simulink model "RefModel_TaskOutput_tmp_backup"  (R2015b)
settings: configuration reference "CenterOutReachConfigSet" (kept outside this file)
undefined symbols (not defined in the file or in its folder): SimulinkParameter_TunableNote
settings Model: Creator=djoshea  LastModifiedBy=shenoylab
settings ConfigSetRef: SourceLocation=Base Workspace

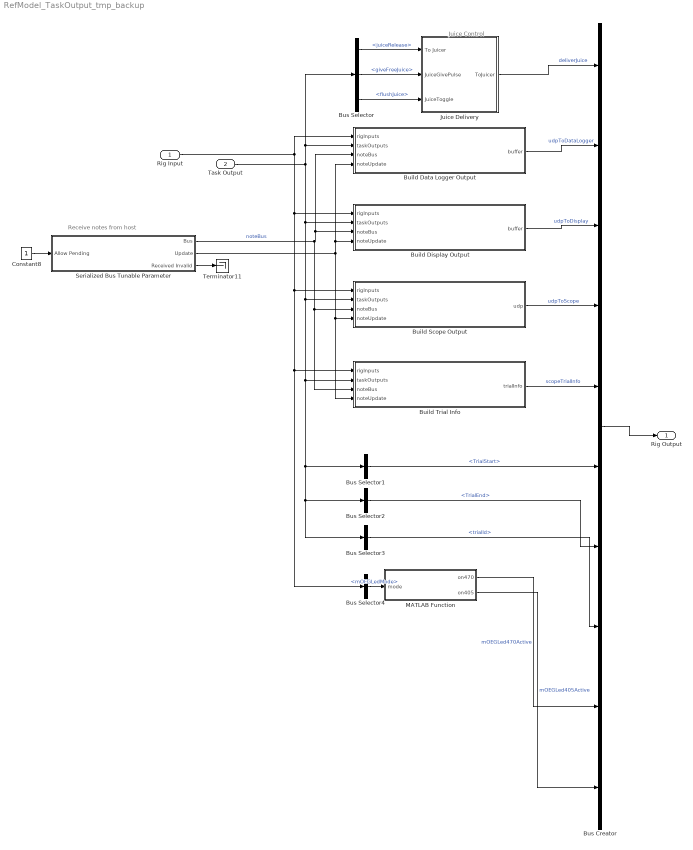
== system RefModel_TaskOutput_tmp_backup ==
  note: Juice Control
  note: Receive notes from host
  Rig Input : Inport  OutDataTypeStr=Bus: RigInputBus  PortDimensions=1  SampleTime=[0.001,0]  Interpolate=off  BusOutputAsStruct=on
  Task Output : Inport  Port=2  OutDataTypeStr=Bus: TaskOutputBus  PortDimensions=1  SampleTime=[0.001,0]  Interpolate=off  BusOutputAsStruct=on
  Build Data Logger Output : MATLAB Function  TreatAsAtomicUnit=on
  Build Display Output : MATLAB Function  TreatAsAtomicUnit=on
  Build Scope Output : MATLAB Function  TreatAsAtomicUnit=on
  Build Trial Info : MATLAB Function  TreatAsAtomicUnit=on
  Bus Creator : BusCreator  Inputs=10  OutDataTypeStr=Bus: RigOutputBus  NonVirtualBus=on
  Bus Selector : BusSelector  OutputSignals=juiceRelease,taskControl.giveFreeJuice,taskControl.flushJuice
  Bus Selector1 : BusSelector  OutputSignals=TrialStart
  Bus Selector2 : BusSelector  OutputSignals=TrialEnd
  Bus Selector3 : BusSelector  OutputSignals=trialId
  Bus Selector4 : BusSelector  OutputSignals=scopeState.mOEGLedMode
  Constant8 : Constant  OutDataTypeStr=uint8
  Juice Delivery : Subsystem
  MATLAB Function : MATLAB Function  TreatAsAtomicUnit=on
  Serialized Bus Tunable Parameter : Subsystem  AncestorBlock=libBusSerialize/Serialized Bus Tunable Parameter  mask(BusSerialize Tunable Parameter Block){paramName='TunableNote'}
      mask prompts: paramName "Parameter Name"
      mask help: This block provides the value of a tunable Simulink.Parameter into the model. Since tunable parameters with xPC target can only be doubles, the functions BusSerialize.createTunableParameter and BusSerialize.setTunableParameter automatically handle typecasting and update counter insertion, and this block handles update detection, typecasting, and reshaping back to the original form. Currently, variable size parameters are not supported.
      mask init:
      | BusSerialize.maskSerializedBusTunableParameterBlockUpdate(gcb);
      mask Display:
      | port_label('output', 1, paramName);
      | port_label('output', 2, 'Update');
      | port_label('output', 3, 'Received Invalid');
      | port_label('input', 1, 'Allow Pending');
  Terminator11 : Terminator
  Rig Output : Outport  OutDataTypeStr=Bus: RigOutputBus  PortDimensions=1  SampleTime=[0.001,0]  BusOutputAsStruct=on
  wires:
  Rig Input/1 -> Build Trial Info/1(rigInputs), Bus Selector4/1, Build Scope Output/1(rigInputs), Build Display Output/1(rigInputs), Build Data Logger Output/1(rigInputs)
  Bus Creator/1 -> Rig Output/1
  Build Data Logger Output/1(buffer) -> Bus Creator/2  "udpToDataLogger"
  Build Display Output/1(buffer) -> Bus Creator/3  "udpToDisplay"
  Bus Selector/2 -> Juice Delivery/2(JuiceGivePulse)  "<giveFreeJuice>"
  Bus Selector/1 -> Juice Delivery/1(To Juicer)  "<juiceRelease>"
  Bus Selector/3 -> Juice Delivery/3(JuiceToggle)  "<flushJuice>"
  Juice Delivery/1(ToJuicer) -> Bus Creator/1  "deliverJuice"
  Constant8/1 -> Serialized Bus Tunable Parameter/1(Allow Pending)
  Serialized Bus Tunable Parameter/3(Received Invalid) -> Terminator11/1
  Serialized Bus Tunable Parameter/1(Bus) -> Build Trial Info/3(noteBus), Build Scope Output/3(noteBus), Build Data Logger Output/3(noteBus), Build Display Output/3(noteBus)  "noteBus"
  Bus Selector1/1 -> Bus Creator/6  "<TrialStart>"
  Serialized Bus Tunable Parameter/2(Update) -> Build Trial Info/4(noteUpdate), Build Scope Output/4(noteUpdate), Build Data Logger Output/4(noteUpdate), Build Display Output/4(noteUpdate)
  Build Scope Output/1(udp) -> Bus Creator/4  "udpToScope"
  Bus Selector2/1 -> Bus Creator/7  "<TrialEnd>"
  Task Output/1 -> Build Data Logger Output/2(taskOutputs), Bus Selector/1, Build Scope Output/2(taskOutputs), Build Trial Info/2(taskOutputs), Bus Selector3/1, Bus Selector2/1, Bus Selector1/1, Build Display Output/2(taskOutputs)
  Bus Selector3/1 -> Bus Creator/8  "<trialId>"
  Bus Selector4/1 -> MATLAB Function/1(mode)  "<mOEGLedMode>"
  MATLAB Function/2(on405) -> Bus Creator/10  "mOEGLed405Active"
  MATLAB Function/1(on470) -> Bus Creator/9  "mOEGLed470Active"
  Build Trial Info/1(trialInfo) -> Bus Creator/5  "scopeTrialInfo"

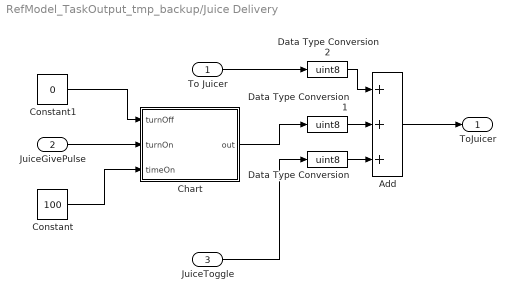
== system RefModel_TaskOutput_tmp_backup/Juice Delivery ==
  To Juicer : Inport
  JuiceGivePulse : Inport  Port=2
  JuiceToggle : Inport  Port=3
  Add : Sum  Inputs=+++
  Chart : Stateflow chart  TreatAsAtomicUnit=on
  Constant : Constant  Value=100  OutDataTypeStr=uint32
  Constant1 : Constant  Value=0  OutDataTypeStr=uint8
  Data Type Conversion : DataTypeConversion  OutDataTypeStr=uint8
  Data Type Conversion1 : DataTypeConversion  OutDataTypeStr=uint8
  Data Type Conversion2 : DataTypeConversion  OutDataTypeStr=uint8
  ToJuicer : Outport
  wires:
  Data Type Conversion2/1 -> Add/1
  Data Type Conversion1/1 -> Add/2
  Data Type Conversion/1 -> Add/3
  Constant1/1 -> Chart/1(turnOff)
  JuiceToggle/1 -> Data Type Conversion/1
  Add/1 -> ToJuicer/1
  Constant/1 -> Chart/3(timeOn)
  JuiceGivePulse/1 -> Chart/2(turnOn)
  Chart/1(out) -> Data Type Conversion1/1
  To Juicer/1 -> Data Type Conversion2/1

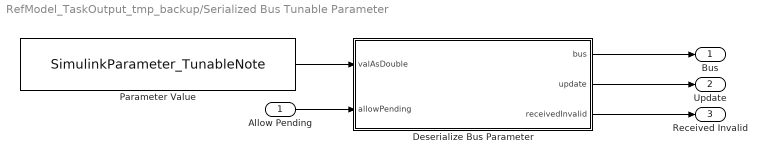
== system RefModel_TaskOutput_tmp_backup/Serialized Bus Tunable Parameter ==
  Allow Pending : Inport
  Deserialize Bus Parameter : MATLAB Function  TreatAsAtomicUnit=on
  Parameter Value : Constant  Value=SimulinkParameter_TunableNote  OutDataTypeStr=double
  Bus : Outport  PortDimensions=1
  Update : Outport  Port=2  OutDataTypeStr=uint8  PortDimensions=1
  Received Invalid : Outport  Port=3  OutDataTypeStr=uint8  PortDimensions=1
  wires:
  Parameter Value/1 -> Deserialize Bus Parameter/1(valAsDouble)
  Allow Pending/1 -> Deserialize Bus Parameter/2(allowPending)
  Deserialize Bus Parameter/3(receivedInvalid) -> Received Invalid/1
  Deserialize Bus Parameter/1(bus) -> Bus/1
  Deserialize Bus Parameter/2(update) -> Update/1

== matlab function RefModel_TaskOutput_tmp_backup/Build Scope Output ==
  data: udp output uint8 size=RigInfo.outputSizes.udpToScope; rigInputs input Bus: RigInputBus size=1; taskOutputs input Bus: TaskOutputBus size=1; noteBus input Bus: NoteBus size=1; noteUpdate input uint8 size=1; RigInfo parameter size=1
function udp  = buildScopeOutput(rigInputs, taskOutputs, noteBus, noteUpdate, RigInfo)
%#codegen

    coder.cinclude('<stdlib.h>'); % for sprintf

    coder.varsize('udp', RigInfo.outputSizes.udpToScope);
    coder.varsize('trialInfo', RigInfo.outputSizes.trialInfoToScope);
    
    bHeader = uint8('#D')';
    bTrialId = uint32(taskOutputs.trialId);
    bConditionId = uint16(taskOutputs.condition.conditionId);
    bSaveNextFrame = uint8(taskOutputs.trialData.saveNextFrame);
    bImageDecoderTraining = uint8(taskOutputs.param.imageDecoderTraining);
    
    udp = [bHeader; bTrialId; bConditionId; bSaveNextFrame; bImageDecoderTraining];
    
    
    
    if ~isempty(udp)
        % add null-terminator for udp and make sure byte count is even,
        % needed for Windows, not sure why
        if mod(numel(udp), 2) == 0
            udp = [udp; uint8(' '); uint8(0)];
        else
            udp = [udp; uint8(0)];
        end
    end
    
end








%     
%     bEmpty = zeros(0, 1, 'uint8');
%     
%     persistent pImagingActive;
%     if isempty(pImagingActive)
%         pImagingActive = uint8(0);
%     end
%     
%     % initialize trigger to zero
%     trigger = uint8(0);
%     
%     % initialize tokens to empty
%     maxNextTrial = 500;
%     coder.varsize('bNextTrial', maxNextTrial);
%     bNextTrial = bEmpty;
%     
%     maxStartImaging = 20;
%     coder.varsize('bStartImaging', maxStartImaging);
%     bStartImaging = bEmpty;
%     
%     maxStopImaging = 20;
%     coder.varsize('bStopImaging', maxStopImaging);
%     bStopImaging = bEmpty;
%     
%     trialInfo = bEmpty;
% 
%     % serialize scope commands
%     if taskOutputs.taskControl.controlImaging && ~isempty(taskOutputs.scopeCommandQueue)
%         % loop through scope commands and generate the command text for
%         % each 
%         coder.varsize('bNextTrial', maxNextTrial);
%         for i = 1:numel(taskOutputs.scopeCommandQueue)
%             command = taskOutputs.scopeCommandQueue(i);
%             
%             switch command
%                 case ScopeCommand.NextTrial
%                     buffer = zeros(maxNextTrial, 1, 'uint8');
%                     nBytes = int32(0);
%                     % can't use %s with sprintf reliably, believe it has to
%                     % do with uint8 vecs as inputs not being necessarily
%                     % null-terminated like strings. You need to use
%                     % coder.rref if you try it
%                     nBytes = coder.ceval('sprintf', coder.ref(buffer), ...
%                         ['NextTrial trialID=%d, dataStore=' taskOutputs.dataLoggerInfo.dataStore' ...
%                         ', subject=' taskOutputs.dataLoggerInfo.subject' ...
%                         ', protocol=' taskOutputs.dataLoggerInfo.protocol' ';' uint8(0)], ...
%                         taskOutputs.trialId);
%                  %   coder.ceval('printf', [char('Scope: next trial command') 10 0]);                        
%                     
%                     if nBytes > maxNextTrial
%                         bNextTrial = buffer(1:maxNextTrial);
%                     else
%                         bNextTrial = buffer(1:nBytes);
%                     end
%                     
%                     % also generate a command to send to the PrairieView
%                     % voltage recording
%                     trialInfoBuffer = zeros(RigInfo.outputSizes.trialInfoToScope, 1, 'uint8');
%                     nBytes = coder.ceval('sprintf', coder.ref(trialInfoBuffer), ...
%                         ['id=%d,c=%d,d=' enumToString_DirectionName(taskOutputs.condition.targetDirectionName)' ';' uint8(0)], ...
%                         taskOutputs.trialId, taskOutputs.condition.conditionId);
%                      if nBytes > RigInfo.outputSizes.trialInfoToScope
%                          trialInfo = trialInfoBuffer(1:RigInfo.outputSizes.trialInfoToScope);
%                      else
%                          trialInfo = trialInfoBuffer(1:nBytes);
%                      end
%                          
%                 case ScopeCommand.StartImagingOnTrigger
%                     % will start t-series if not already in one
%                    % coder.ceval('printf', [char('Scope: sending start imaging command') 10 0]);                        
%                     bStartImaging = uint8('StartImaging;')';
%                     
%                 case ScopeCommand.StartTrialImaging
%                     % send trigger to start trial
%                     if ~pImagingActive
%                         pImagingActive = uint8(1);
%                         coder.ceval('printf', [char('Scope: sending start trial trigger') 10 0]);
%                         trigger = uint8(1);
%                     end
%                     
%                 case ScopeCommand.EndTrialImaging
%                     % send trigger to stop trial
%                     if pImagingActive
%                         pImagingActive = uint8(0);
%                         %coder.ceval('printf', [char('Scope: sending end trial trigger') 10 0]);
%                         %trigger = uint8(1);
%                     end
%                     
%                 case ScopeCommand.StopImaging
%                     % will stop t-series
%                     bStopImaging = uint8('StopImaging;')';
%             end
%         end
%     end
%     
%     if pImagingActive && ~taskOutputs.taskControl.controlImaging
%         % shut down imaging since we're no longer controlling it
%         bStopImaging = uint8('StopImaging;')';
%     end
%     
%     udp = [bNextTrial; bStartImaging; bStopImaging];

== matlab function RefModel_TaskOutput_tmp_backup/MATLAB Function ==
  data: mode input Enum: LedMode size=1; on470 output uint8 size=1; on405 output uint8 size=1
function [on470, on405] = getLedStatus(mode)
%#codegen

    on470 = uint8(0);
    on405 = uint8(0);
    
    switch mode
        case LedMode.Off
            
        case LedMode.CW405
            on405 = uint8(1);

        case LedMode.CW470
            on470 = uint8(1);
    
        case LedMode.Alternating405_470
            on470 = uint8(1);
            on405 = uint8(1);
    end
end

== matlab function RefModel_TaskOutput_tmp_backup/Build Trial Info ==
  data: trialInfo output uint8 size=RigInfo.outputSizes.udpToScope; rigInputs input Bus: RigInputBus size=1; taskOutputs input Bus: TaskOutputBus size=1; noteBus input Bus: NoteBus size=1; noteUpdate input uint8 size=1; RigInfo parameter size=1
function trialInfo  = buildScopeTrialInfo(rigInputs, taskOutputs, noteBus, noteUpdate, RigInfo)
%#codegen

    coder.cinclude('<stdlib.h>'); % for sprintf

    coder.varsize('udp', RigInfo.outputSizes.udpToScope);
    coder.varsize('trialInfo', RigInfo.outputSizes.trialInfoToScope);
   
    
    bEmpty = zeros(0, 1, 'uint8');
    
%     persistent pImagingActive;
%     if isempty(pImagingActive)
%         pImagingActive = uint8(0);
%     end
%     
%     % initialize trigger to zero
%     trigger = uint8(0);
%     
%     % initialize tokens to empty
%     maxNextTrial = 500;
%     coder.varsize('bNextTrial', maxNextTrial);
%     bNextTrial = bEmpty;
%     
%     maxStartImaging = 20;
%     coder.varsize('bStartImaging', maxStartImaging);
%     bStartImaging = bEmpty;
%     
%     maxStopImaging = 20;
%     coder.varsize('bStopImaging', maxStopImaging);
%     bStopImaging = bEmpty;
    
    trialInfo = bEmpty;

    % serialize scope commands
    if taskOutputs.taskControl.controlImaging && ~isempty(taskOutputs.scopeCommandQueue)
        % loop through scope commands and generate the command text for
        % each 
%         coder.varsize('bNextTrial', maxNextTrial);
        for i = 1:numel(taskOutputs.scopeCommandQueue)
            command = taskOutputs.scopeCommandQueue(i);
            
            switch command
                case ScopeCommand.NextTrial
%                     buffer = zeros(maxNextTrial, 1, 'uint8');
%                     nBytes = int32(0);
%                     % can't use %s with sprintf reliably, believe it has to
%                     % do with uint8 vecs as inputs not being necessarily
%                     % null-terminated like strings. You need to use
%                     % coder.rref if you try it
%                     nBytes = coder.ceval('sprintf', coder.ref(buffer), ...
%                         ['NextTrial trialID=%d, dataStore=' taskOutputs.dataLoggerInfo.dataStore' ...
%                         ', subject=' taskOutputs.dataLoggerInfo.subject' ...
%                         ', protocol=' taskOutputs.dataLoggerInfo.protocol' ';' uint8(0)], ...
%                         taskOutputs.trialId);
%                  %   coder.ceval('printf', [char('Scope: next trial command') 10 0]);                        
%                     
%                     if nBytes > maxNextTrial
%                         bNextTrial = buffer(1:maxNextTrial);
%                     else
%                         bNextTrial = buffer(1:nBytes);
%                     end
                    
                    % also generate a command to send to the PrairieView
                    % voltage recording
                    trialInfoBuffer = zeros(RigInfo.outputSizes.trialInfoToScope, 1, 'uint8');
                    nBytes = coder.ceval('sprintf', coder.ref(trialInfoBuffer), ...
                        ['id=%d,c=%d,d=' enumToString_DirectionName(taskOutputs.condition.targetDirectionName)' ';' uint8(0)], ...
                        taskOutputs.trialId, taskOutputs.condition.conditionId);
                     if nBytes > RigInfo.outputSizes.trialInfoToScope
                         trialInfo = trialInfoBuffer(1:RigInfo.outputSizes.trialInfoToScope);
                     else
                         trialInfo = trialInfoBuffer(1:nBytes);
                     end
                         
%                 case ScopeCommand.StartImagingOnTrigger
%                     % will start t-series if not already in one
%                    % coder.ceval('printf', [char('Scope: sending start imaging command') 10 0]);                        
%                     bStartImaging = uint8('StartImaging;')';
%                     
%                 case ScopeCommand.StartTrialImaging
%                     % send trigger to start trial
%                     if ~pImagingActive
%                         pImagingActive = uint8(1);
%                         coder.ceval('printf', [char('Scope: sending start trial trigger') 10 0]);
%                         trigger = uint8(1);
%                     end
%                     
%                 case ScopeCommand.EndTrialImaging
%                     % send trigger to stop trial
%                     if pImagingActive
%                         pImagingActive = uint8(0);
%                         %coder.ceval('printf', [char('Scope: sending end trial trigger') 10 0]);
%                         %trigger = uint8(1);
%                     end
%                     
%                 case ScopeCommand.StopImaging
%                     % will stop t-series
%                     bStopImaging = uint8('StopImaging;')';
            end
        end
    end
    
%     if pImagingActive && ~taskOutputs.taskControl.controlImaging
%         % shut down imaging since we're no longer controlling it
%         bStopImaging = uint8('StopImaging;')';
%     end
    
%     udp = [bNextTrial; bStartImaging; bStopImaging];

    
    
end

== stateflow chart RefModel_TaskOutput_tmp_backup/Juice Delivery/Chart ==
  state On
    en:
    out = uint8(1);
    ex:
    out = uint8(0);
  state Waiting
  (default) -> Waiting
  Waiting -> On : [turnOn==1]
  On -> Waiting [order 1] : after(timeOn, tick)
  On -> Waiting [order 2] : [turnOff==1]
  data: turnOff input uint8 size=1; turnOn input uint8 size=1; timeOn input uint32 size=1; out output uint8 size=1

== matlab function RefModel_TaskOutput_tmp_backup/Serialized Bus Tunable Parameter/Deserialize Bus Parameter ==
  data: valAsDouble input double; bus output Bus: NoteBus size=1; update output uint8 size=1; allowPending input uint8 size=1; receivedInvalid output uint8 size=1
function [bus, update, receivedInvalid] = deserializeBusParameter(valAsDouble, allowPending)
%#codegen

    % typecast to bytes
    valAsBytes = typecast(valAsDouble, 'uint8');

    % use the first byte as updateCounter, check for whether counter has been incremented
    thisCounter = valAsBytes(1);
    persistent pLastCounter;
    if isempty(pLastCounter)
        pLastCounter = thisCounter;
    end
    if pLastCounter ~= thisCounter
        recvUpdate = uint8(1);
        pLastCounter = thisCounter;
    else
        recvUpdate = uint8(0);
    end
    startOffset = 2;

    % external cached output for when allowPending 
    persistent pBusOut;
    if isempty(pBusOut)
        pBusOut = initializeBus_NoteBus();
    end

    % parse incoming bytes if allowing updates
    receivedInvalid = uint8(0);
    if allowPending
        [bus, valid] = deserializeBus_NoteBus(valAsBytes, startOffset);
        if valid
            % update internal cache
            pBusOut = bus;
        else
            % don't update internal cache, output internal cache
            bus = pBusOut;
            receivedInvalid = uint8(1);
            recvUpdate = uint8(0);
        end
    else
        bus = pBusOut;
    end

    % track whether we have a pending update
    persistent pPending;
    if isempty(pPending), pPending = uint8(0); end
    if recvUpdate
        if allowPending
            % update goes out immediately
            update = uint8(1);
            pPending = uint8(0);
        else
            % queue pending update
            update = uint8(0);
            pPending = uint8(1);
        end
    else
        if allowPending
            % release pending
            update = pPending;
            pPending = uint8(0);
        else
            % do nothing
            update = uint8(0);
        end
    end

    % reset fields marked with .resetImmediately immediately after update
    if ~update

    end
end

== matlab function RefModel_TaskOutput_tmp_backup/Build Data Logger Output ==
  data: buffer output uint8 size=RigInfo.outputSizes.udpToDataLogger; rigInputs input; taskOutputs input; noteBus input Bus: NoteBus size=1; noteUpdate input uint8 size=1; RigInfo parameter
function buffer = buildDataLoggerOutput(rigInputs, taskOutputs, noteBus, noteUpdate, RigInfo)
%#codegen

bEmpty = zeros(0, 1, 'uint8');
coder.varsize('buffer', RigInfo.outputSizes.udpToDataLogger);
buffer = zeros(0, 1, 'uint8');

if taskOutputs.taskControl.saveData && taskOutputs.taskControl.runTask && ~taskOutputs.trialData.inPurgatory

    % timestamp for data logger
    timestamp = rigInputs.clock;

    % send TrialStart info
    if taskOutputs.TrialStart
        % send data logger info
        bDataInfo = serializeBusWithDataLoggerHeader_DataLoggerInfoBus(...
            taskOutputs.dataLoggerInfo, BusSerialize.GroupTypes.Control, uint8('info'), timestamp);

        % send next trial with new trial id
        % once TrialStart goes high, the trialId field has already updated
        nextTrialBus = initializeBus_DataLoggerNextTrialBus();
        nextTrialBus.nextTrial = taskOutputs.trialId;
        bNextTrial = serializeBusWithDataLoggerHeader_DataLoggerNextTrialBus(...
            nextTrialBus, BusSerialize.GroupTypes.Control, uint8('nextTrial'), timestamp);

        % send this trial's parameters
        bParam = serializeBusWithDataLoggerHeader_ParamBus(...
            taskOutputs.param, BusSerialize.GroupTypes.Parameter, uint8('param'), timestamp);

        % send this trial's condition
        bCondition = serializeBusWithDataLoggerHeader_ConditionBus(...
            taskOutputs.condition, BusSerialize.GroupTypes.Parameter, uint8('condition'), timestamp);
    else
        bDataInfo = bEmpty;
        bNextTrial = bEmpty;
        bParam = bEmpty;
        bCondition = bEmpty;
    end
    
    if taskOutputs.TrialITI
        % send TrialDataOutputBus
        bTrialData = serializeBusWithDataLoggerHeader_TrialDataOutputBus(...
            taskOutputs.trialDataOutput, BusSerialize.GroupTypes.Parameter, uint8('trialData'), timestamp);
        
        % send MicroscopeStateBus
        bScopeState = serializeBusWithDataLoggerHeader_MicroscopeStateBus(...
            rigInputs.scopeState, BusSerialize.GroupTypes.Parameter, uint8('scope'), timestamp);
    else
        bTrialData = bEmpty;
        bScopeState = bEmpty;
    end

    % serialize handOutput on handUpdate
    if rigInputs.hand.handUpdate
        bHand = serializeBusWithDataLoggerHeader_HandOutputBus(...
            taskOutputs.handOutput, BusSerialize.GroupTypes.Analog, uint8('hand'), timestamp);
    else
        bHand = bEmpty;
    end
    
    % serialize eyeOutput on eyeUpdate
    if rigInputs.eye.eyeUpdate
        bEye = serializeBusWithDataLoggerHeader_EyeOutputBus(...
            taskOutputs.eyeOutput, BusSerialize.GroupTypes.Analog, uint8('eye'), timestamp);
    else
        bEye = bEmpty;
    end
    
    % serialize analogOutput (every tick)
    bAnalog = serializeBusWithDataLoggerHeader_AnalogOutputBus(...
            taskOutputs.analogOutput, BusSerialize.GroupTypes.Analog, uint8('analog'), timestamp);
        
    % serialize scopeTiming (every tick)
    bScopeTiming = serializeBusWithDataLoggerHeader_ScopeTimingBus(...
            rigInputs.scopeTiming, BusSerialize.GroupTypes.Analog, uint8('scopeTiming'), timestamp);
    
    % serialize mOEGFrameInfo (every tick)
    bmOEGFrameInfo = serializeBusWithDataLoggerHeader_mOEGFrameInfoBus(...
            rigInputs.mOEGFrameInfo, BusSerialize.GroupTypes.Analog, uint8('mOEGFrameInfo'), timestamp);
        
    % serialize scope events
    coder.varsize('bScopeEvents', 1000, 1);
    bScopeEvents = bEmpty;
    scopeEventBus = initializeBus_ScopeEventBus();
    if rigInputs.scopeTiming.cameraFrameEnd
        scopeEventBus.event = ScopeEvent.CameraFrameEnd;
        bScopeEvents = [bScopeEvents; serializeBusWithDataLoggerHeader_ScopeEventBus(...
            scopeEventBus, BusSerialize.GroupTypes.Event, uint8('scopeEvent'), timestamp)];
    end
        
    % serialize noteBus on update
    if noteUpdate
        bNote = serializeBusWithDataLoggerHeader_NoteBus(...
            noteBus, BusSerialize.GroupTypes.Note, uint8('note'), timestamp);
    else
        bNote = bEmpty;
    end

    coder.varsize('bTaskEvents', 1000, 1);
    bTaskEvents = bEmpty;
    eventBus = initializeBus_TaskEventBus();
    for i = 1:numel(taskOutputs.taskEventQueue)
        eventBus.event = taskOutputs.taskEventQueue(i);
        bTaskEvents = [bTaskEvents; serializeBusWithDataLoggerHeader_TaskEventBus(...
            eventBus, BusSerialize.GroupTypes.Event, uint8('taskEvent'), timestamp)]; %#ok<AGROW>
    end
    
    buffer = [bDataInfo; bNextTrial; bParam; bCondition; bTrialData; bScopeState; ...
        bHand; bEye; bAnalog; bScopeTiming; bScopeEvents; bmOEGFrameInfo; bNote; bTaskEvents];
end

end

== matlab function RefModel_TaskOutput_tmp_backup/Build Display Output ==
  data: buffer output uint8 size=RigInfo.outputSizes.udpToDisplay; rigInputs input; taskOutputs input; noteBus input Bus: NoteBus size=1; noteUpdate input uint8 size=1; RigInfo parameter
function buffer = buildDisplayOutput(rigInputs, taskOutputs, noteBus, noteUpdate, RigInfo)
%#codegen

    coder.varsize('buffer', RigInfo.outputSizes.udpToDisplay);
    bEmpty = zeros(0, 1, 'uint8');

    % timestamp for data logger
    timestamp = rigInputs.clock;

    % send TrialStart info
    if taskOutputs.TrialStart
        % send data logger info
        bDataInfo = serializeBusWithDataLoggerHeader_DataLoggerInfoBus(...
            taskOutputs.dataLoggerInfo, BusSerialize.GroupTypes.Control, uint8('info'), timestamp);

        % send next trial with new trial id
        nextTrialBus = initializeBus_DataLoggerNextTrialBus();
        nextTrialBus.nextTrial = taskOutputs.trialId;
        bNextTrial = serializeBusWithDataLoggerHeader_DataLoggerNextTrialBus(...
            nextTrialBus, BusSerialize.GroupTypes.Control, uint8('nextTrial'), timestamp);

        % send this trial's parameters
        bParam = serializeBusWithDataLoggerHeader_ParamBus(...
            taskOutputs.param, BusSerialize.GroupTypes.Parameter, uint8('P'), timestamp);

        % send this trial's condition
        bCondition = serializeBusWithDataLoggerHeader_ConditionBus(...
            taskOutputs.condition, BusSerialize.GroupTypes.Parameter, uint8('C'), timestamp);

        % set display task
        busSetTask = initializeBus_DisplaySetTaskBus();
        busSetTask.taskName = uint8('CenterOutReachTask');
        busSetTask.taskVersion = uint32(20150121);
        bSetTask = serializeBusWithDataLoggerHeader_DisplaySetTaskBus(...
            busSetTask, BusSerialize.GroupTypes.Parameter, uint8('setTask'), timestamp);
    else
        bDataInfo = bEmpty;
        bNextTrial = bEmpty;
        bParam = bEmpty;
        bCondition = bEmpty;
        bSetTask = bEmpty;
    end

    % serialize task commands
    if ~isempty(taskOutputs.displayCommandQueue)
        coder.varsize('bCommand', 10000);
        % send trialData before each group of taskCommands
        bCommand = serializeBusWithDataLoggerHeader_TrialDataBus(...
            taskOutputs.trialData, BusSerialize.GroupTypes.Parameter, uint8('trialData'), timestamp);

        % loop through task commands and serialize them, crucial that this
        % be analog
        commandBus = initializeBus_DisplayCommandBus();
        for i = 1:numel(taskOutputs.displayCommandQueue)
            commandBus.taskCommand = taskOutputs.displayCommandQueue(i);
            bCommand = [bCommand; serializeBusWithDataLoggerHeader_DisplayCommandBus(...
                commandBus, BusSerialize.GroupTypes.Analog, uint8('taskCommand'), timestamp)]; %#ok<AGROW>
        end
    else
        bCommand = bEmpty;
    end

    % serialize handOutput if updated as Param
    if rigInputs.hand.handUpdate
        bHand = serializeBusWithDataLoggerHeader_HandOutputBus(...
            taskOutputs.handOutput, BusSerialize.GroupTypes.Parameter, uint8('handInfo'), timestamp);
    else
        bHand = bEmpty;
    end

    % serialize noteBus on update
    if noteUpdate
        bNote = serializeBusWithDataLoggerHeader_NoteBus(...
            noteBus, BusSerialize.GroupTypes.Note, uint8('note'), timestamp);
    else
        bNote = bEmpty;
    end

    % assemble the final output
    buffer = [bDataInfo; bNextTrial; bParam; bCondition; bSetTask; bCommand; bHand; bNote];

end
